simulink model "Filter_module"  (R2018a)
settings: Solver=VariableStepAuto  StartTime=0.0  StopTime=1  RelTol=1e-3
settings Model: Creator=HP  LastModifiedBy=HP

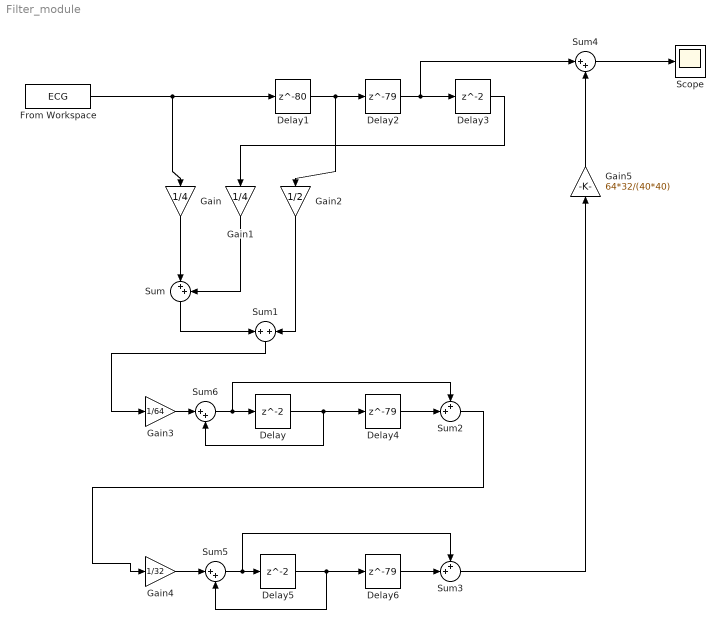
== system Filter_module ==
  Delay : Delay  InitialCondition=0
  Delay1 : Delay  DelayLength=80  InitialCondition=0
  Delay2 : Delay  DelayLength=79  InitialCondition=0
  Delay3 : Delay  InitialCondition=0
  Delay4 : Delay  DelayLength=79  InitialCondition=0
  Delay5 : Delay  InitialCondition=0
  Delay6 : Delay  DelayLength=79  InitialCondition=0
  From Workspace : FromWorkspace  VariableName=ECG  SampleTime=0
  Gain : Gain  Gain=1/4
  Gain1 : Gain  Gain=1/4
  Gain2 : Gain  Gain=1/2
  Gain3 : Gain  Gain=1/64
  Gain4 : Gain  Gain=1/32
  Gain5 : Gain  Gain=64*32/(40*40)
  Scope : Scope
  Sum{,4..6} (4 alike) : Sum  Inputs=|++
  Sum1 : Sum
  Sum2 : Sum  Inputs=++|
  Sum3 : Sum  Inputs=++|
  wires:
  Delay1/1 -> Gain2/1, Delay2/1
  Gain1/1 -> Sum/2
  Gain/1 -> Sum/1
  Gain2/1 -> Sum1/2
  Sum/1 -> Sum1/1
  Sum1/1 -> Gain3/1
  Delay4/1 -> Sum2/2
  Delay6/1 -> Sum3/2
  Sum2/1 -> Gain4/1
  Gain5/1 -> Sum4/2
  Delay3/1 -> Gain1/1
  Gain4/1 -> Sum5/1
  Gain3/1 -> Sum6/1
  Sum5/1 -> Sum3/1, Delay5/1
  Sum6/1 -> Sum2/1, Delay/1
  Delay/1 -> Sum6/2, Delay4/1
  Delay5/1 -> Sum5/2, Delay6/1
  Sum3/1 -> Gain5/1
  Delay2/1 -> Sum4/1, Delay3/1
  Sum4/1 -> Scope/1
  From Workspace/1 -> Gain/1, Delay1/1
